simulink model "Junctions4"  (Simulink 6.0)
settings: Solver=ode45  StartTime=0.0  StopTime=10.0  RelTol=1e-3
settings Model: Creator=scaife  LastModifiedBy=scaife  ExtModeAutoUpdateStatusClock=off
settings DataIOCC: SignalLoggingName=sigsOut
settings DebuggingCC: SolverPrmCheckMsg=none
settings HardwareCC: TargetUnknown=on
settings STFCustomTargetCC: TargetFcnLib=ansi_tfl_tmw.mat  GenFloatMathFcnCalls=ANSI_C  ModelReferenceCompliant=off  SystemTargetFile=grt.tlc

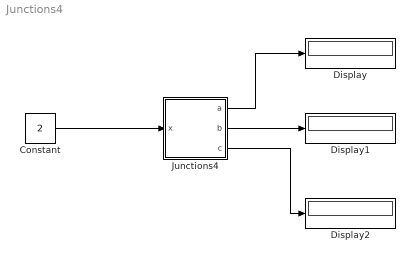
== system Junctions4 ==
  Constant : Constant  Value=2
  Display : Display
  Display1 : Display
  Display2 : Display
  Junctions4 : Stateflow chart
  wires:
  Junctions4/1(a) -> Display/1
  Junctions4/2(b) -> Display1/1
  Junctions4/3(c) -> Display2/1
  Constant/1 -> Junctions4/1(x)

== stateflow chart Junctions4 ==
  state TOP
    state A/
      en:c+=1
      ex:c+=10
    state B/
      en:c+=100
      du:c+=1000
    A -> (junction 6) : [x<4]{a+=100}
    A -> (junction 6) : [x>=4]{a+=1000}
    (junction 6) -> B : [x%%3==1]
        | {a+=100000}
        | /b+=100000
    (default) -> A : [x<>0]{a+=10}/b+=10
    (default) -> A : [x==0]{a+=1}/b+=1
    (junction 6) -> B : [x%%3==0]
        | {a+=10000}
        | /b+=10000
    B -> TOP
  (default) -> TOP
  data: x input int32; a output int32 =111111; b output int32 =111111; c output int32 =111111
